simulink model "simulinkMonkey"  (R2019b)
settings: Solver=VariableStepAuto  StartTime=0.0  StopTime=10.0  RelTol=1e-3
values from neighbouring files (symbols this model uses):
  q0 = [0; 0; pi/2]    [Monkey3Link_Fixed_mrt.m]    (also in Monkey3Link_SM_mrt.m = [0; pi/2; 0; -l1 - l3/2; 0]; simulateM_mkd.m = [-pi/12; -pi/12; pi/12; pi/12; pi/12]; simulateSM_mkd.m = [pi/2; -pi/2; -0.3; -0.45; 0])
settings Model: Creator=Mike Dermksian  LastModifiedBy=Mike Dermksian

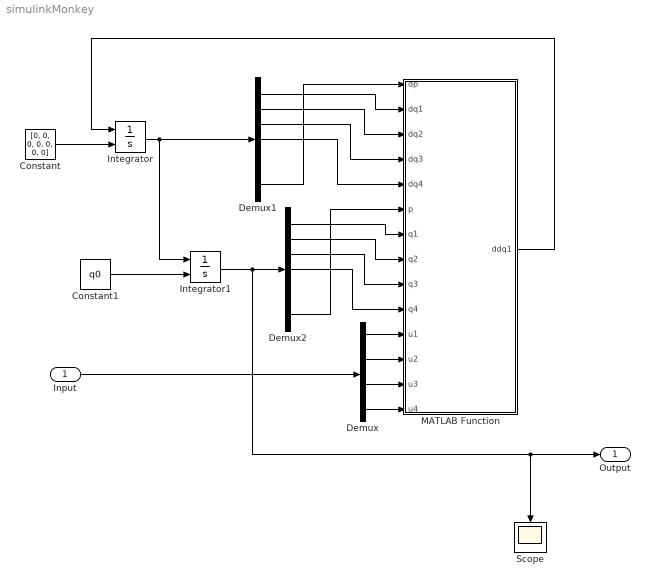
== system simulinkMonkey ==
  Input : Inport
  Constant : Constant  Value=[0, 0, 0, 0, 0, 0, 0]
  Constant1 : Constant  Value=q0
  Demux : Demux
  Demux1 : Demux  Outputs=7
  Demux2 : Demux  Outputs=7
  Integrator : Integrator  InitialConditionSource=external
  Integrator1 : Integrator  InitialConditionSource=external
  MATLAB Function : MATLAB Function  TreatAsAtomicUnit=on
  Scope : Scope
  Output : Outport
  wires:
  Integrator/1 -> Demux1/1, Integrator1/1
  MATLAB Function/1(ddq1) -> Integrator/1
  Demux1/7 -> MATLAB Function/1(dp)
  Demux1/1 -> MATLAB Function/2(dq1)
  Demux1/2 -> MATLAB Function/3(dq2)
  Demux1/3 -> MATLAB Function/4(dq3)
  Demux1/4 -> MATLAB Function/5(dq4)
  Demux2/1 -> MATLAB Function/7(q1)
  Integrator1/1 -> Output/1, Scope/1, Demux2/1
  Demux2/2 -> MATLAB Function/8(q2)
  Demux2/3 -> MATLAB Function/9(q3)
  Demux2/7 -> MATLAB Function/6(p)
  Demux2/4 -> MATLAB Function/10(q4)
  Input/1 -> Demux/1
  Demux/1 -> MATLAB Function/11(u1)
  Demux/2 -> MATLAB Function/12(u2)
  Demux/3 -> MATLAB Function/13(u3)
  Demux/4 -> MATLAB Function/14(u4)
  Constant/1 -> Integrator/2
  Constant1/1 -> Integrator1/2

== matlab function simulinkMonkey/MATLAB Function ==
  data: dp input; ddq1 output; dq1 input; dq2 input; dq3 input; dq4 input; p input; q1 input; q2 input; q3 input; q4 input; u1 input; u2 input; u3 input; u4 input
function ddq1 = fcn(dp,dq1,dq2,dq3,dq4,p,q1,q2,q3,q4,u1,u2,u3,u4)
ddq1 = simulinkDynamics(dp,dq1,dq2,dq3,dq4,p,q1,q2,q3,q4,u1,u2,u3,u4);
